simulink model "dve_nadrze_rizeni"  (R2020a)
settings: Solver=VariableStepAuto  StartTime=0.0  StopTime=300.0  RelTol=1e-3
settings Model: Creator=Filip Jašek  LastModifiedBy=Filip Jašek

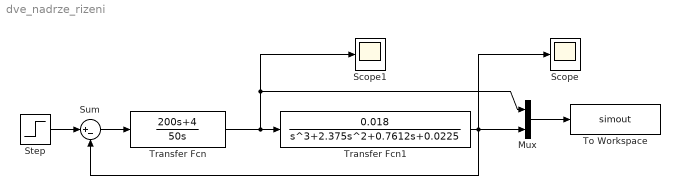
== system dve_nadrze_rizeni ==
  Mux : Mux  Inputs=2
  Scope : Scope
  Scope1 : Scope
  Step : Step  Time=0  SampleTime=0
  Sum : Sum  Inputs=|+-
  To Workspace : ToWorkspace  VariableName=simout  SaveFormat=Timeseries  SampleTime=-1
  Transfer Fcn : TransferFcn  Numerator=[200,4]  Denominator=[50,0]
  Transfer Fcn1 : TransferFcn  Numerator=[0.018]  Denominator=[1,2.375,0.7612,0.0225]
  wires:
  Transfer Fcn/1 -> Mux/1, Scope1/1, Transfer Fcn1/1
  Transfer Fcn1/1 -> Sum/2, Mux/2, Scope/1
  Step/1 -> Sum/1
  Sum/1 -> Transfer Fcn/1
  Mux/1 -> To Workspace/1
